simulink model "Lab2_SimulinkFinal"  (R2023a)
settings: Solver=VariableStepAuto  StartTime=0.0  StopTime=20  RelTol=1e-3
values from neighbouring files (symbols this model uses):
  A = [-0.4 1 0; -4 0 40; 0 0 -4]    [Ejemplo.m]
  B = [0; 0; 2]    [Ejemplo.m]
  C = [1 0 0]    [Ejemplo.m]
  D = [0]    [Ejemplo.m]
  x0 = [0.34 0 0]'    [Ejemplo.m]
settings Model: Creator=syaba  LastModifiedBy=syaba

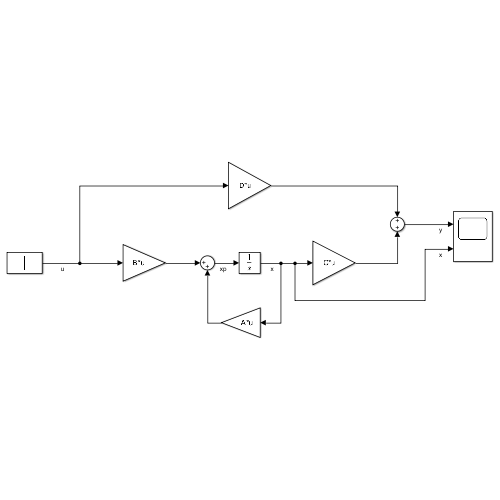
[thumbnail: Simulink's stored preview of the top-level diagram]
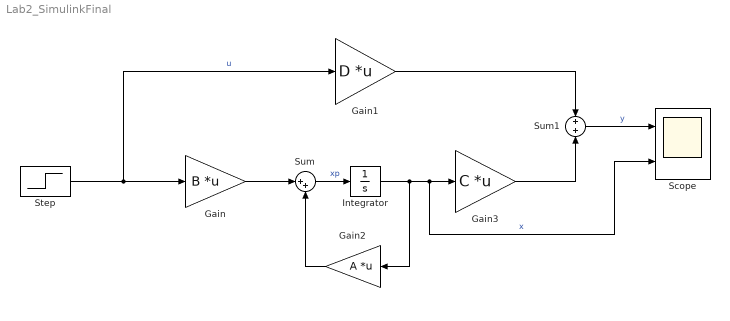
== system Lab2_SimulinkFinal ==
  Gain : Gain  Gain=B  Multiplication=Matrix(K*u)
  Gain1 : Gain  Gain=D  Multiplication=Matrix(K*u)
  Gain2 : Gain  Gain=A  Multiplication=Matrix(K*u)
  Gain3 : Gain  Gain=C  Multiplication=Matrix(K*u)
  Integrator : Integrator  InitialCondition=x0
  Scope : Scope  NumInputPorts=2
  Step : Step  Time=0  After=0  SampleTime=0.01
  Sum : Sum  Inputs=|++
  Sum1 : Sum
  wires:
  Step/1 -> Gain1/1, Gain/1  "u"
  Gain/1 -> Sum/1
  Gain2/1 -> Sum/2
  Sum/1 -> Integrator/1  "xp"
  Integrator/1 -> Scope/2, Gain3/1, Gain2/1  "x"
  Gain1/1 -> Sum1/1
  Gain3/1 -> Sum1/2
  Sum1/1 -> Scope/1  "y"
